simulink model "LAB4_primoEs"  (R2025b)
settings: Solver=ode45  StartTime=0.0  StopTime=Tend  MaxStep=0.001*Ts  MinStep=0.0001*Ts  RelTol=1e-3
undefined symbols (not defined in the file): C, K, Ts
libraries: cstblocks x1
settings Model: Creator=davidecovolo  LastModifiedBy=davidecovolo
settings SolverCC: InitialStep=0.0001*Ts

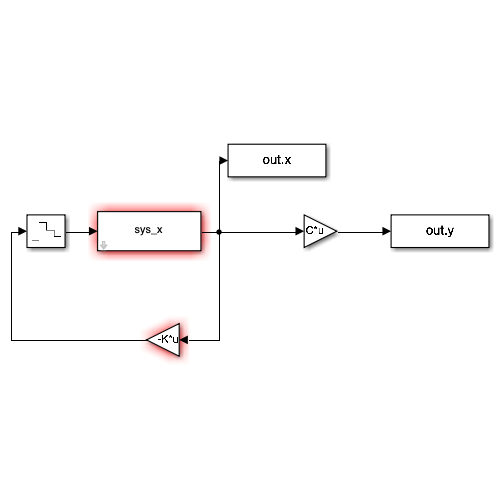
[thumbnail: Simulink's stored preview of the top-level diagram]
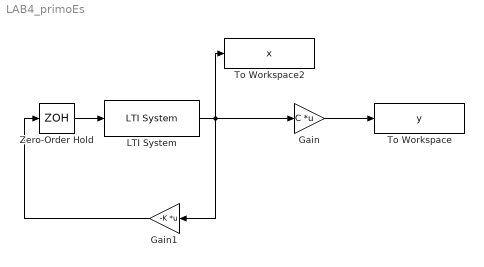
== system LAB4_primoEs ==
  Gain : Gain  Gain=C  Multiplication=Matrix(K*u)
  Gain1 : Gain  Gain=-K  Multiplication=Matrix(K*u)
  LTI System : cstblocks/LTI System  sys=sys_x  IC=x0  PadeOrder=0
  To Workspace : ToWorkspace  VariableName=y  SaveFormat=Timeseries  SampleTime=Ts
  To Workspace2 : ToWorkspace  VariableName=x  SaveFormat=Timeseries  SampleTime=Ts
  Zero-Order Hold : ZeroOrderHold  SampleTime=Ts
  wires:
  Zero-Order Hold/1 -> LTI System/1
  Gain1/1 -> Zero-Order Hold/1
  Gain/1 -> To Workspace/1
  LTI System/1 -> To Workspace2/1, Gain/1, Gain1/1
